simulink model "power_reference_2"  (R2021a)
settings: Solver=ode4  StartTime=0.0  StopTime=60*60*24  FixedStep=1e-2  RelTol=1e-3
undefined symbols (not defined in the file): i, P, P_n, pc1, pc2, pc3, pc4, pc5, Vnominal
settings Model: Creator=Usuario  LastModifiedBy=pedro
settings SolverCC: AlgebraicLoopSolver=TrustRegion
settings DataIOCC: SaveOutput=off  SignalLogging=off  DSMLogging=off  SaveTime=off  ReturnWorkspaceOutputs=off
settings DebuggingCC: SFMachineParentedDataDiag=warning

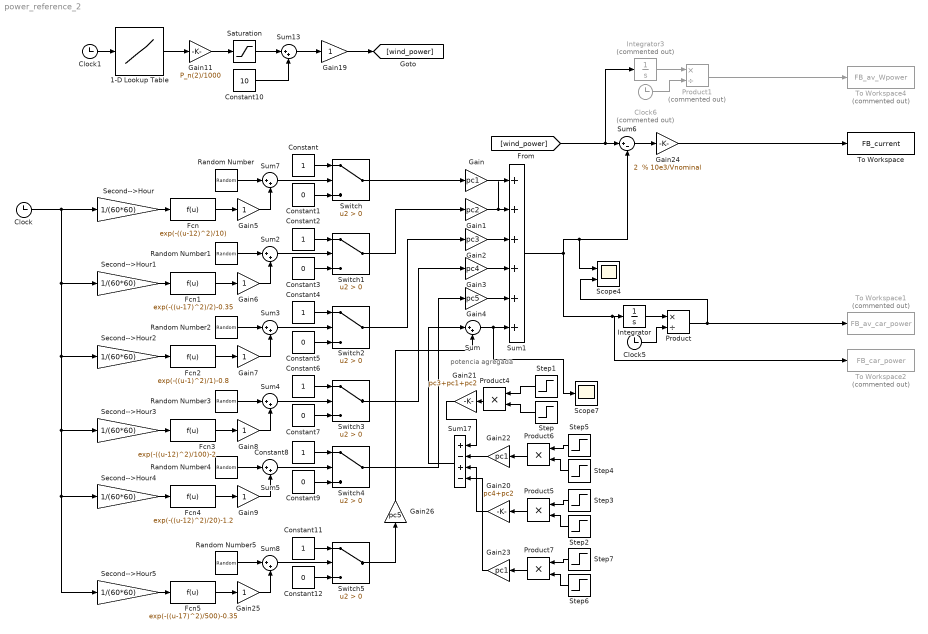
== system power_reference_2 ==
  note: potencia agregada
  1-D Lookup Table : Lookup_n-D  NumberOfTableDimensions=1  BreakpointsForDimension1=P(i).time  Table=P(i).signals.values  InterpMethod=Cubic spline  InternalRulePriority=Speed  RndMeth=Simplest  InputSameDT=on
  Clock : Clock
  Clock1 : Clock
  Clock5 : Clock
  Clock6 : Clock  Commented=on
  Constant{,2,4,6,8,11} (6 alike) : Constant
  Constant{1,3,5,7,9,12} (6 alike) : Constant  Value=0
  Constant10 : Constant  Value=10
  Fcn : Fcn  Expr=exp(-((u-12)^2)/10)
  Fcn1 : Fcn  Expr=exp(-((u-17)^2)/2)-0.35
  Fcn2 : Fcn  Expr=exp(-((u-1)^2)/1)-0.8
  Fcn3 : Fcn  Expr=exp(-((u-12)^2)/100)-2
  Fcn4 : Fcn  Expr=exp(-((u-12)^2)/20)-1.2
  Fcn5 : Fcn  Expr=exp(-((u-17)^2)/500)-0.35
  Gain : Gain  Gain=pc1
  Gain1 : Gain  Gain=pc2
  Gain11 : Gain  Gain=P_n(2)/1000
  Gain{5..9,19,25} (7 alike) : Gain
  Gain2 : Gain  Gain=pc3
  Gain20 : Gain  Gain=pc4+pc2
  Gain21 : Gain  Gain=pc3+pc1+pc2
  Gain22 : Gain  Gain=pc1
  Gain23 : Gain  Gain=pc1
  Gain24 : Gain  Gain="2  % 10e3/Vnominal"
  Gain26 : Gain  Gain=pc5
  Gain3 : Gain  Gain=pc4
  Gain4 : Gain  Gain=pc5
  Integrator : Integrator
  Integrator3 : Integrator  Commented=on
  Product : Product  Inputs=*/
  Product1 : Product  Commented=on  Inputs=*/
  Product{4..7} (4 alike) : Product
  Random Number{,1..5} (6 alike) : RandomNumber  Seed=1  SampleTime=20*60
  Saturation : Saturate  UpperLimit=P_n(2)/1000  LowerLimit=5
  Scope4 : Scope  NumInputPorts=2
  Scope7 : Scope
  Second-->Hour{,1..5} (6 alike) : Gain  Gain=1/(60*60)
  Step : Step  Time=7*60*60+20*60  SampleTime=0
  Step1 : Step  Time=9*60*60+20*60  Before=1  After=0  SampleTime=0
  Step2 : Step  Time=9*60*60+40*60  SampleTime=0
  Step3 : Step  Time=10*60*60+20*60  Before=1  After=0  SampleTime=0
  Step4 : Step  Time=10*60*60+20*60  SampleTime=0
  Step5 : Step  Time=11*60*60+20*60  Before=1  After=0  SampleTime=0
  Step6 : Step  Time=12*60*60  SampleTime=0
  Step7 : Step  Time=12*60*60+20*60  Before=1  After=0  SampleTime=0
  Sum{,2..5,7..8,13} (8 alike) : Sum  Inputs=|++
  Sum1 : Sum  Inputs=++++++
  Sum17 : Sum  Inputs=+-+-
  Sum6 : Sum  Inputs=|+-
  Switch{,1..5} (6 alike) : Switch  Criteria=u2 > Threshold
  To Workspace : ToWorkspace  VariableName=FB_current  SaveFormat=Structure With Time  SampleTime=-1
  To Workspace1 : ToWorkspace  Commented=on  VariableName=FB_av_car_power  SaveFormat=Structure With Time  SampleTime=-1
      settings: Decimation=10
  To Workspace2 : ToWorkspace  Commented=on  VariableName=FB_car_power  SaveFormat=Structure With Time  SampleTime=-1
      settings: Decimation=10
  To Workspace4 : ToWorkspace  Commented=on  VariableName=FB_av_Wpower  SaveFormat=Structure With Time  SampleTime=-1
  wires:
  Random Number/1 -> Sum7/1
  Constant/1 -> Switch/1
  Constant1/1 -> Switch/3
  Switch/1 -> Gain/1
  Sum7/1 -> Switch/2
  Fcn/1 -> Gain5/1
  Clock/1 -> Second-->Hour4/1, Second-->Hour5/1, Second-->Hour3/1, Second-->Hour2/1, Second-->Hour1/1, Second-->Hour/1
  Second-->Hour/1 -> Fcn/1
  Gain5/1 -> Sum7/2
  Gain/1 -> Sum1/1
  Gain1/1 -> Sum1/2
  Gain2/1 -> Sum1/3
  Gain3/1 -> Sum1/4
  Gain4/1 -> Sum1/5
  Sum2/1 -> Switch1/2
  Switch1/1 -> Gain1/1
  Constant3/1 -> Switch1/3
  Constant2/1 -> Switch1/1
  Gain6/1 -> Sum2/2
  Fcn1/1 -> Gain6/1
  Random Number1/1 -> Sum2/1
  Second-->Hour1/1 -> Fcn1/1
  Sum1/1 -> To Workspace2/1, Integrator/1, Scope4/1, Sum6/2
  Second-->Hour2/1 -> Fcn2/1
  Random Number2/1 -> Sum3/1
  Fcn2/1 -> Gain7/1
  Gain7/1 -> Sum3/2
  Constant4/1 -> Switch2/1
  Constant5/1 -> Switch2/3
  Switch2/1 -> Gain2/1
  Sum3/1 -> Switch2/2
  Sum4/1 -> Switch3/2
  Switch3/1 -> Gain3/1
  Constant7/1 -> Switch3/3
  Constant6/1 -> Switch3/1
  Gain8/1 -> Sum4/2
  Fcn3/1 -> Gain8/1
  Random Number3/1 -> Sum4/1
  Second-->Hour3/1 -> Fcn3/1
  Second-->Hour4/1 -> Fcn4/1
  Random Number4/1 -> Sum5/1
  Fcn4/1 -> Gain9/1
  Gain9/1 -> Sum5/2
  Constant8/1 -> Switch4/1
  Constant9/1 -> Switch4/3
  Sum5/1 -> Switch4/2
  Switch4/1 -> Gain4/1
  [wind_power] -> Integrator3/1, Sum6/1
  Gain24/1 -> To Workspace/1
  Integrator/1 -> Product/1
  Clock5/1 -> Product/2
  Product/1 -> Scope4/2, To Workspace1/1
  Constant10/1 -> Sum13/2
  Integrator3/1 -> Product1/1
  Clock6/1 -> Product1/2
  Product1/1 -> To Workspace4/1
  Gain11/1 -> Saturation/1
  Gain19/1 -> [wind_power]
  Step/1 -> Product4/2
  Step1/1 -> Product4/1
  Step3/1 -> Product5/1
  Step2/1 -> Product5/2
  Product4/1 -> Gain21/1
  Product5/1 -> Gain20/1
  Gain21/1 -> Sum17/1
  Gain20/1 -> Sum17/3
  Sum17/1 -> Sum/1
  Product6/1 -> Gain22/1
  Step4/1 -> Product6/2
  Step5/1 -> Product6/1
  Gain22/1 -> Sum17/2
  Step7/1 -> Product7/1
  Step6/1 -> Product7/2
  Product7/1 -> Gain23/1
  Gain23/1 -> Sum17/4
  Sum6/1 -> Gain24/1
  Sum/1 -> Scope7/1, Sum1/6
  Second-->Hour5/1 -> Fcn5/1
  Random Number5/1 -> Sum8/1
  Fcn5/1 -> Gain25/1
  Gain25/1 -> Sum8/2
  Constant11/1 -> Switch5/1
  Constant12/1 -> Switch5/3
  Sum8/1 -> Switch5/2
  Switch5/1 -> Gain26/1
  Gain26/1 -> Sum/2
  Saturation/1 -> Sum13/1
  Sum13/1 -> Gain19/1
  Clock1/1 -> 1-D Lookup Table/1
  1-D Lookup Table/1 -> Gain11/1
